simulink model "FinalProject2022"  (R2023a)
settings: Solver=ode1be  StartTime=0.0  StopTime=10  RelTol=1e-3
settings Model: Creator=romav  LastModifiedBy=romav

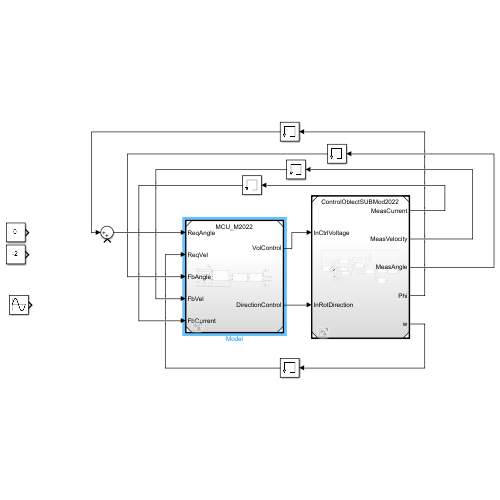
[thumbnail: Simulink's stored preview of the top-level diagram]
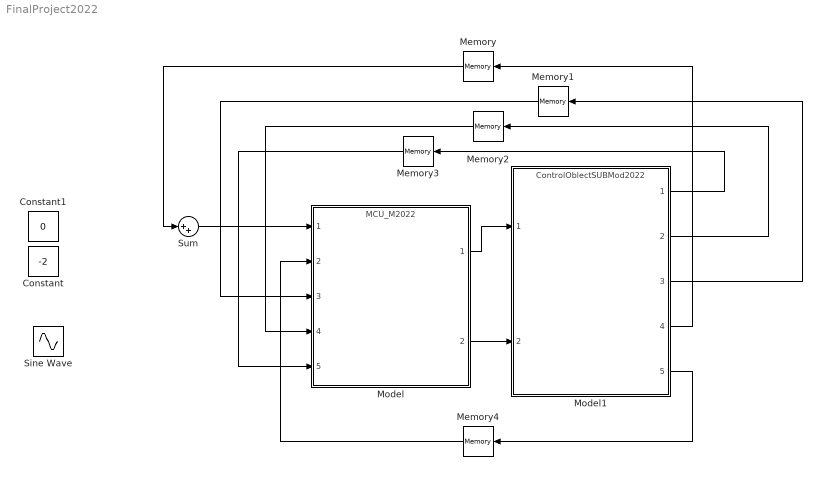
== system FinalProject2022 ==
  Constant : Constant  Value=-2
  Constant1 : Constant  Value=0
  Memory{,1..4} (5 alike) : Memory
  Model : ModelReference  ModelNameDialog=MCU_M2022.slx  SimulationMode=Normal  ModelReferenceVersion=2.0
  Model1 : ModelReference  ModelNameDialog=ControlOblectSUBMod2022.slx  SimulationMode=Normal  ModelReferenceVersion=1.0
  Sine Wave : Sin  SampleTime=0
  Sum : Sum  Inputs=|++
  wires:
  Model/1 -> Model1/1
  Model/2 -> Model1/2
  Model1/1 -> Memory3/1
  Model1/2 -> Memory2/1
  Model1/3 -> Memory1/1
  Model1/4 -> Memory/1
  Model1/5 -> Memory4/1
  Memory/1 -> Sum/1
  Memory1/1 -> Model/3
  Memory2/1 -> Model/4
  Memory3/1 -> Model/5
  Memory4/1 -> Model/2
  Sum/1 -> Model/1
